simulink model "RDGPI_TraditionalPID"  (R2023b)
settings: Solver=VariableStepAuto  StartTime=0.0  StopTime=10.0  RelTol=1e-3
libraries: slpidlib x1
settings Model: Creator=jia  LastModifiedBy=jia

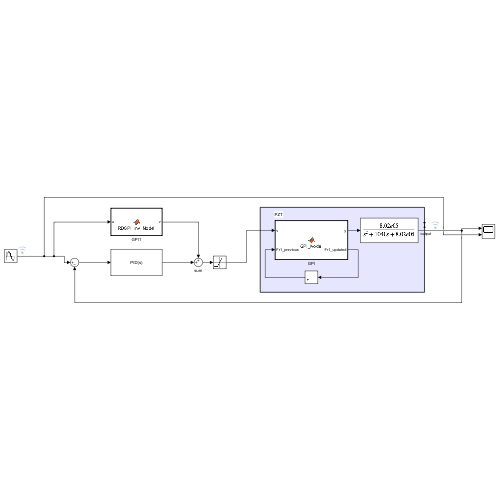
[thumbnail: Simulink's stored preview of the top-level diagram]
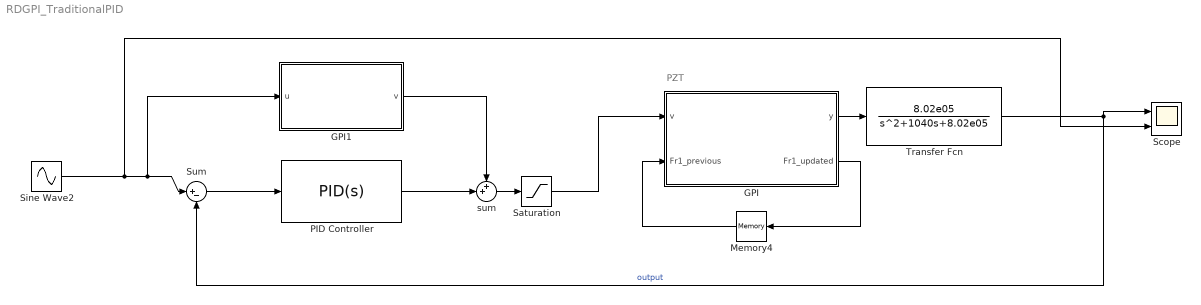
== system RDGPI_TraditionalPID ==
  note: PZT
  GPI : MATLAB Function  TreatAsAtomicUnit=on
  GPI1 : MATLAB Function  TreatAsAtomicUnit=on
  Memory4 : Memory  InheritSampleTime=on  LinearizeMemory=on  LinearizeAsDelay=on
  PID Controller : slpidlib/PID Controller  Controller=PID  Form=Parallel  TimeDomain=Continuous-time  UseExternalTs=off  SampleTime=-1  IntegratorMethod=Forward Euler  FilterMethod=Forward Euler  ControllerParametersSource=internal  P=10.4381021267155  I=4697.59826404073  UseKiTs=off  D=0.00575155798021087  N=405735.272161233  UseFilter=on  TunerSelectOption=Transfer Function Based (PID Tuner App)  InitialConditionSource=internal  InitialConditionForIntegrator=0  InitialConditionForFilter=0  DifferentiatorICPrevScaledInput=0  ExternalReset=none  TrackingMode=off  Kt=1  LimitOutput=off  SatLimitsSource=internal  UpperSaturationLimit=inf  LowerSaturationLimit=-inf  LinearizeAsGain=on  AntiWindupMode=none  Kb=1  LimitIntegrator=off  UpperIntegratorSaturationLimit=inf  LowerIntegratorSaturationLimit=-inf  POutMin=[]  POutMax=[]  IOutMin=[]  IOutMax=[]  DOutMin=[]  DOutMax=[]  NOutMin=[]  NOutMax=[]  SumOutMin=[]  SumOutMax=[]  SaturationOutMin=[]  SaturationOutMax=[]  PParamMin=[]  PParamMax=[]  IParamMin=[]  IParamMax=[]  DParamMin=[]  DParamMax=[]  NParamMin=[]  NParamMax=[]  KbParamMin=[]  KbParamMax=[]  KtParamMin=[]  KtParamMax=[]  KbOutMin=[]  KbOutMax=[]  KtOutMin=[]  KtOutMax=[]  IntegratorOutMin=[]  IntegratorOutMax=[]  FilterOutMin=[]  FilterOutMax=[]  SumI1OutMin=[]  SumI1OutMax=[]  SumI2OutMin=[]  SumI2OutMax=[]  SumI3OutMin=[]  SumI3OutMax=[]  SumI4OutMin=[]  SumI4OutMax=[]  SumDOutMin=[]  SumDOutMax=[]  DifferentiatorOutMin=[]  DifferentiatorOutMax=[]  FilterDiffOutCoefMin=[]  FilterDiffOutCoefMax=[]  ReciprocalOutMin=[]  ReciprocalOutMax=[]  SumDenOutMin=[]  SumDenOutMax=[]  SumNumOutMin=[]  SumNumOutMax=[]  DivideOutMin=[]  DivideOutMax=[]  UdiffTsProdOutMin=[]  UdiffTsProdOutMax=[]  NTsProdOutMin=[]  NTsProdOutMax=[]  UintegralTsProdOutMin=[]  UintegralTsProdOutMax=[]  UngainTsProdOutMin=[]  UngainTsProdOutMax=[]  ClampingZeroOutDataTypeStr=Inherit: Inherit via back propagation  ClampingZeroOutMin=[]  ClampingZeroOutMax=[]  FilterDenConstantOutDataTypeStr=Inherit: Inherit via back propagation  FilterDenConstantOutMin=[]  FilterDenConstantOutMax=[]  PCopyOutDataTypeStr=Inherit: Inherit via back propagation  PCopyOutMin=[]  PCopyOutMax=[]  NCopyOutDataTypeStr=Inherit: Inherit via back propagation  NCopyOutMin=[]  NCopyOutMax=[]  IntegratorContinuousStateAttributes=''  IntegratorStateMustResolveToSignalObject=off  IntegratorRTWStateStorageClass=Auto  FilterContinuousStateAttributes=''  FilterStateMustResolveToSignalObject=off  FilterRTWStateStorageClass=Auto  ParallelPVariant=InternalParameters  IdealPVariant=Disabled  IVariant=InternalParameters  DVariant=InternalParameters  IntegratorVariant=Continuous  SatVariant=Disabled  AWVariant=Passthrough  PCopyVariant=Disabled  TRVariant=Disabled  FdbkBlocksVariant=Forward  IdealPFdbkVariant=Disabled  SatFdbkVariant=Disabled  DerivativeFilterVariant=ContFilter  NVariant=InternalParameters  NCopyVariant=Disabled  FilterICVariant=InternalICsFilter  IntegratorICVariant=InternalICs  ExternalResetVariant=Disabled  TRSumVariant=Passthrough  SumFdbkVariant=Disabled  SumVariant=Sum_PID  TsampFilterVariant=InternalTs  TsampNgainVariant=Passthrough  TsampIntegralVariant=Disabled_SignalSpec  ExternalSaturationOutDataTypeStr=Inherit: Same as second input
  Saturation : Saturate  UpperLimit=10  LowerLimit=0
  Scope : Scope  NumInputPorts=2
  Sine Wave2 : Sin  Amplitude=2  Bias=2.5  Frequency=2*pi  SampleTime=0.0001
  Sum : Sum  Inputs=|+-
  Transfer Fcn : TransferFcn  Numerator=[8.02e05]  Denominator=[1 1040 8.02e05]
  sum : Sum  Inputs=++|
  wires:
  GPI/1(y) -> Transfer Fcn/1
  GPI/2(Fr1_updated) -> Memory4/1
  Memory4/1 -> GPI/2(Fr1_previous)
  sum/1 -> Saturation/1
  Transfer Fcn/1 -> Sum/2, Scope/1  "output"
  Sum/1 -> PID Controller/1
  Sine Wave2/1 -> Scope/2, GPI1/1(u), Sum/1
  GPI1/1(v) -> sum/1
  Saturation/1 -> GPI/1(v)
  PID Controller/1 -> sum/2

== matlab function RDGPI_TraditionalPID/GPI1 ==
  data: u input; v output
function v = RDGPI_Inv_Model(u)
    %20250804
    rd = [ -0.50 0.00 0.15 0.30 0.60 1.20 2.40 4.80 ];
    eta = [ 0.000100 0.383196 0.006316 0.056768 0.021432 -0.174859 -0.044040 -0.025427 ];
    P = [ 2.125828 1.019777 0.296430 0.530357 ];
    tau = [ -0.191598 0.000000 0.057479 0.115906 0.249790 0.530417 0.881841 1.478992 ];
    mu = [ -0.000681 2.609631 -0.042316 -0.326569 -0.102678 1.276615 0.604400 0.457474 ];
    q = [ 0.470405 -0.152501 -0.027378 -0.038788 ];
    m1 = 0.11729583 ;
    m2 = 0.00007254 ;
%% 202507
% rd = [-0.5 0 0.15 0.3 0.6 1.2 2.4 4.8];  % 示例值，需根据实际模型调整
% eta= [0.0001    0.1495    1.2567    0.3082   -1.4465    0.0601   -0.0217   -0.0455];
% P=[3.1004   12.5217  -22.0931    9.6164];
% m1=0.0093;
% m2=7.5072e-04;
% 
% tau = [ -0.074750 0.000000 0.022425 0.233355 0.747675 0.908415 1.302015 2.037135 ];
% mu = [ -0.004471 6.688963 -5.977827 -0.127842 3.149442 -0.683956 0.215993 0.569583 ];
% q = [ 0.322539 -0.258527 -0.218548 0.472460 ];

    dt = 0.0001;
    % 初始化持久变量（仅保存历史状态，无需计算参数）
    persistent first_run Fr2_last u_last
    if isempty(first_run)
        first_run = true;
        Fr2_last = zeros(length(P), 1);  % 初始化play算子历史值
        u_last = 0;                      % 初始化上一步输入
    end
    
    % ------ 逐点实时计算（核心逻辑） ------ %
    % 1. 计算输入变化率dv_dt（当前步与上一步的差分）
    if first_run
        dv_dt = 0;  % 第一步变化率为0
    else
        dv_dt = (u - u_last) / dt;  % 后续步用差分计算
    end
    u_last = u;  % 保存当前输入，用于下一步计算
    % 2. 计算动态阈值r（基于当前dv_dt）
     r = m1 * (0:length(P))' + m2 * abs(dv_dt);  % 与P长度匹配的列向量
    
    % 3. 计算z（play算子中间变量）
    z = zeros(length(P), 1);  % 初始化z为列向量
    z(1) = P(1) * r(1);       % 第一个元素计算
    for i = 2:length(P)
        sum_p = sum(P(1:i));  % 累加P的前i个元素
        z(i) = z(i-1) + sum_p * (r(i) - r(i-1));  % 递推计算z
    end
    
    % 4. PI逆模型：更新play算子Fr2
    Fr2 = zeros(length(P), 1);  % 初始化当前步Fr2
    for j = 1:length(P)
        F_inc = u;                  % 递增方向输入
        F_dec = u;                  % 递减方向输入
        A = F_inc - z(j);           % 递增约束
        B = min(F_dec + z(j), Fr2_last(j));  % 递减约束（结合历史值）
        Fr2(j) = max(A, B);         % 取约束的最大值，更新当前步Fr2
    end
    Fr2_last = Fr2;  % 保存当前Fr2，作为下一步的历史值
    
    % 5. 计算PI逆模型输出x
    x = q * Fr2;  % 用固定q与Fr2相乘（矩阵乘法）
    
    % 6. G逆模型：计算Ad_inv和输出v
    Ad_inv = zeros(length(tau), 1);  % 初始化Ad_inv
    for z_idx = 1:length(tau)
        if tau(z_idx) > 0
            Ad_inv(z_idx) = max(x - tau(z_idx), 0);  % 正阈值激活
        elseif tau(z_idx) < 0
            Ad_inv(z_idx) = min(x - tau(z_idx), 0);  % 负阈值激活
        else
            Ad_inv(z_idx) = x;  % 零阈值直接取x
        end
    end
    v = mu * Ad_inv;  % 用固定mu与Ad_inv相乘，得到G逆模型输出
    
    % 最终输出（逆模型总输出）
    v = v;
end

== matlab function RDGPI_TraditionalPID/GPI ==
  data: v input; Fr1_previous input; y output; Fr1_updated output
function [y,Fr1_updated] = GPI_Model(v, Fr1_previous)
    %% v  % 0-10V,0.001s,1000hz
    
    rd = [-8    -6    -4    -2     0     2     4     6     8];
    eta = [1.0000    1.0000    1.0000    1.0000    1.2437   -0.1103   -0.0787   -0.1742   -0.1767];
    r=[0     1     2     3     4     5];
    n=length(r);
    P=[0.7460    0.1860    0.0650    0.0855    0.0362   -0.1159];

    Ad = zeros(length(rd),1);
    for z = 1:length(rd)
        if rd(z) > 0
            Ad(z) = max(v - rd(z), 0);
        elseif rd(z) < 0
            Ad(z) = min(v - rd(z), 0);
        else
            Ad(z) = v;
        end
    end
    w = eta * Ad;

    Fr1 = zeros(n, 1);
    % 对于每个阈值r(j)，更新Fr1(j)
    for j = 1:n
        if ~isempty(Fr1_previous)
            Fr1(j) = Fr1_previous(j);
        end
        F_inc = w;
        F_dec = w;
        A = F_inc - r(j);
        B = min(F_dec + r(j), Fr1(j));
        Fr1(j) = max(A, B); % Equation (1)
    end
    %% 输出y
    y = P*Fr1;
    Fr1_updated = Fr1;
end
